simulink model "EricNREL5_FF_Pitch_ConstPwr"  (Simulink 7.7)
settings: Solver=ode4  StartTime=0  StopTime=TMax  FixedStep=DT  MaxStep=DT  RelTol=1e-3
undefined symbols (not defined in the file): alpha, DR, DT, FF_dynamicWindSpeed, FF_Time, GenEff, KI, KK, KP, MaxPit, MinPit, NDOF, NumOuts, OutList, PitDotMax, q_init, qdot_init, SSPitch, strmatch, TdotMax, Tmax, Ts, w_rated, wo
settings Model: Creator=dwilso  LastModifiedBy=oooeee
settings DataIOCC: LimitDataPoints=off  SaveOutput=off  SignalLoggingName=sigsOut
settings OptimizationCC: InlineInvariantSignals=on  InitFltsAndDblsToZero=on
settings DebuggingCC: SaveWithParameterizedLinksMsg=none  SignalResolutionControl=TryResolveAllWithWarning  SolverPrmCheckMsg=none  MultiTaskDSMMsg=warning  MultiTaskCondExecSysMsg=none  StrictBusMsg=None
settings HardwareCC: TargetUnknown=on
settings RTWCC: IncludeERTFirstTime=on
settings GRTTargetCC: TargetFcnLib=ansi_tfl_tmw.mat  ModelReferenceCompliant=off  MatFileLogging=off

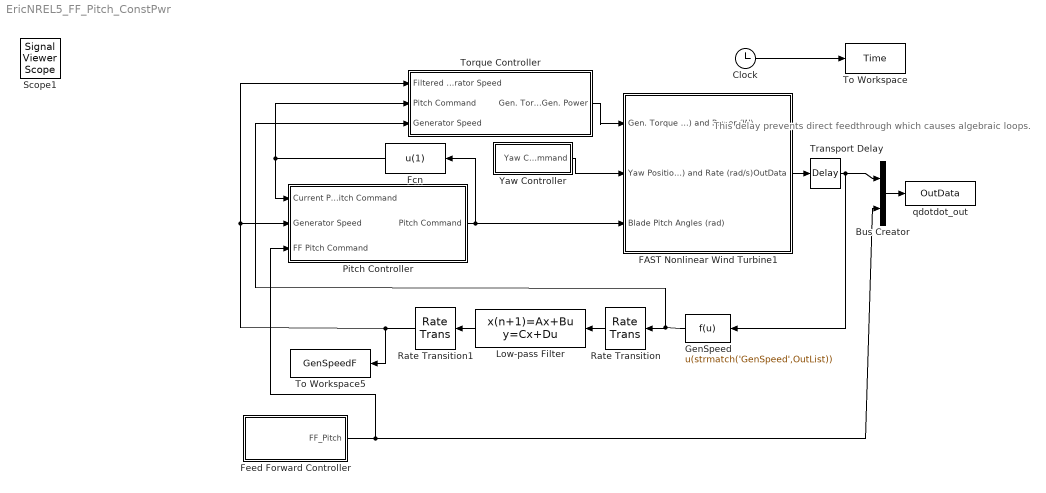
== system EricNREL5_FF_Pitch_ConstPwr ==
  note: This delay prevents direct
      | feedthrough which causes
      |  algebraic loops.
  Bus Creator : BusCreator  Inputs=2
  Clock : Clock
      settings: Decimation=10
  FAST Nonlinear Wind Turbine1 : Subsystem  mask(FAST Nonlinear Wind Turbine){}
      mask help: This block contains the FAST S-Function and blocks that integrate the DOF accelerations to get velocities and displacements.
      mask init:
      | clear FAST_SFunc
  Fcn : Fcn  Expr=u(1)
  Feed Forward Controller : Subsystem
  GenSpeed : Fcn  Expr=u(strmatch('GenSpeed',OutList))
  Low-pass Filter : DiscreteStateSpace  A=alpha  B=1-alpha  C=alpha  D=1-alpha  X0=728.47  SampleTime=Ts
  Pitch Controller : Subsystem
  Rate Transition : RateTransition  OutPortSampleTime=Ts
  Rate Transition1 : RateTransition
  To Workspace : ToWorkspace  VariableName=Time  SampleTime=DT  SaveFormat=Array
  To Workspace5 : ToWorkspace  VariableName=GenSpeedF  SampleTime=-1  SaveFormat=Array
  Torque Controller : Subsystem
  Transport Delay : TransportDelay  DelayTime=.00001
  Yaw Controller : Subsystem
  qdotdot_out : ToWorkspace  VariableName=OutData  SampleTime=DT  SaveFormat=Array
  Scope1 : SignalViewerScope  IOType=viewer  ZoomMode=xonly  RefreshTime=0.035000
  wires:
  Clock/1 -> To Workspace/1
  Yaw Controller/1(Yaw Command) -> FAST Nonlinear Wind Turbine1/2(Yaw Position (rad) and Rate (rad/s))
  GenSpeed/1 -> Rate Transition/1, Torque Controller/3(Generator Speed)
  Low-pass Filter/1 -> Rate Transition1/1
  Fcn/1 -> Pitch Controller/1(Current Pitch Command), Torque Controller/2(Pitch Command)
  Rate Transition/1 -> Low-pass Filter/1
  Rate Transition1/1 -> Torque Controller/1(Filtered Generator Speed), Pitch Controller/2(Generator Speed), To Workspace5/1
  Bus Creator/1 -> qdotdot_out/1
  FAST Nonlinear Wind Turbine1/1(OutData) -> Transport Delay/1
  Transport Delay/1 -> Bus Creator/1, GenSpeed/1
  Torque Controller/1("Gen. Torque,  Gen. Power") -> FAST Nonlinear Wind Turbine1/1(Gen. Torque (Nm) and Power (W))
  Pitch Controller/1(Pitch Command) -> FAST Nonlinear Wind Turbine1/3(Blade Pitch Angles (rad)), Fcn/1
  Feed Forward Controller/1(FF_Pitch) -> Bus Creator/2, Pitch Controller/3(FF Pitch Command)

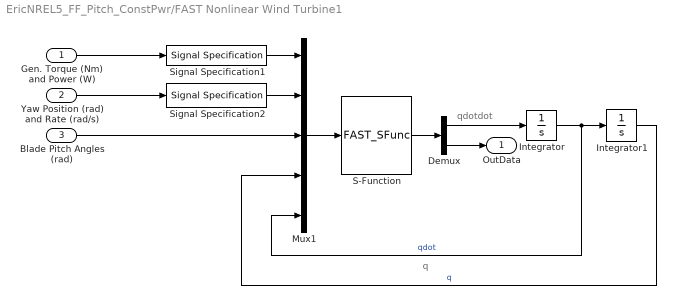
== system EricNREL5_FF_Pitch_ConstPwr/FAST Nonlinear Wind Turbine1 ==
  note: qdotdot
  note: q
  Gen. Torque (Nm) and Power (W) : Inport
  Yaw Position (rad) and Rate (rad/s) : Inport  Port=2
  Blade Pitch Angles (rad) : Inport  Port=3
  Demux : Demux  Outputs=[NDOF, NumOuts]
  Integrator : Integrator  InitialCondition=qdot_init
  Integrator1 : Integrator  InitialCondition=q_init
  Mux1 : Mux  Inputs=5
  S-Function : S-Function  FunctionName=FAST_SFunc  EnableBusSupport=off
  Signal Specification1 : SignalSpecification  OutDataTypeStr=double  Dimensions=2
  Signal Specification2 : SignalSpecification  OutDataTypeStr=double  Dimensions=2
  OutData : Outport
  wires:
  Integrator/1 -> Integrator1/1, Mux1/5  "qdot"
  Gen. Torque (Nm) and Power (W)/1 -> Signal Specification1/1
  S-Function/1 -> Demux/1
  Demux/1 -> Integrator/1
  Demux/2 -> OutData/1
  Mux1/1 -> S-Function/1
  Blade Pitch Angles (rad)/1 -> Mux1/3
  Yaw Position (rad) and Rate (rad/s)/1 -> Signal Specification2/1
  Integrator1/1 -> Mux1/4  "q"
  Signal Specification1/1 -> Mux1/1
  Signal Specification2/1 -> Mux1/2

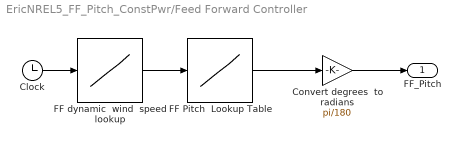
== system EricNREL5_FF_Pitch_ConstPwr/Feed Forward Controller ==
  Clock : Clock
      settings: Decimation=10
  Convert degrees  to radians : Gain  Gain=pi/180
  FF Pitch  Lookup Table : Lookup  InputValues=SSPitch(:,1)  Table=SSPitch(:,2)
  FF dynamic  wind  speed lookup : Lookup  InputValues=FF_Time  Table=FF_dynamicWindSpeed
  FF_Pitch : Outport
  wires:
  FF Pitch  Lookup Table/1 -> Convert degrees  to radians/1
  FF dynamic  wind  speed lookup/1 -> FF Pitch  Lookup Table/1
  Clock/1 -> FF dynamic  wind  speed lookup/1
  Convert degrees  to radians/1 -> FF_Pitch/1

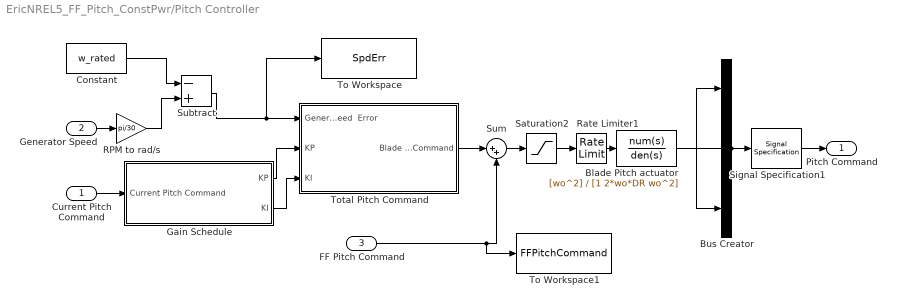
== system EricNREL5_FF_Pitch_ConstPwr/Pitch Controller ==
  Current Pitch Command : Inport
  Generator Speed : Inport  Port=2
  FF Pitch Command : Inport  Port=3
  Blade Pitch actuator : TransferFcn  Numerator=[wo^2]  Denominator=[1 2*wo*DR wo^2]
  Bus Creator : BusCreator  Inputs=3
  Constant : Constant  Value=w_rated
  Gain Schedule : Subsystem
  RPM to rad/s : Gain  Gain=pi/30  SaturateOnIntegerOverflow=on  OutDataTypeStr=Inherit: Same as input  ParamDataTypeStr=Inherit: Same as input
  Rate Limiter1 : RateLimiter  RisingSlewLimit=PitDotMax  FallingSlewLimit=-PitDotMax  SampleTimeMode=inherited
  Saturation2 : Saturate  UpperLimit=MaxPit  LowerLimit=MinPit
  Signal Specification1 : SignalSpecification  OutDataTypeStr=double  Dimensions=3
  Subtract : Sum  Inputs=-+
  Sum : Sum  Inputs=|++
  To Workspace : ToWorkspace  VariableName=SpdErr  SampleTime=-1  SaveFormat=Array
  To Workspace1 : ToWorkspace  VariableName=FFPitchCommand  SampleTime=-1  SaveFormat=Array
  Total Pitch Command : Subsystem
  Pitch Command : Outport
  wires:
  Constant/1 -> Subtract/1
  Bus Creator/1 -> Signal Specification1/1
  Signal Specification1/1 -> Pitch Command/1
  Generator Speed/1 -> RPM to rad/s/1
  Current Pitch Command/1 -> Gain Schedule/1(Current Pitch Command)
  Gain Schedule/1(KP) -> Total Pitch Command/2(KP)
  Gain Schedule/2(KI) -> Total Pitch Command/3(KI)
  Subtract/1 -> Total Pitch Command/1(Generator Speed  Error), To Workspace/1
  RPM to rad/s/1 -> Subtract/2
  Blade Pitch actuator/1 -> Bus Creator/3, Bus Creator/2, Bus Creator/1
  Total Pitch Command/1(Blade Pitch Command) -> Sum/1
  Sum/1 -> Saturation2/1
  FF Pitch Command/1 -> Sum/2, To Workspace1/1
  Saturation2/1 -> Rate Limiter1/1
  Rate Limiter1/1 -> Blade Pitch actuator/1

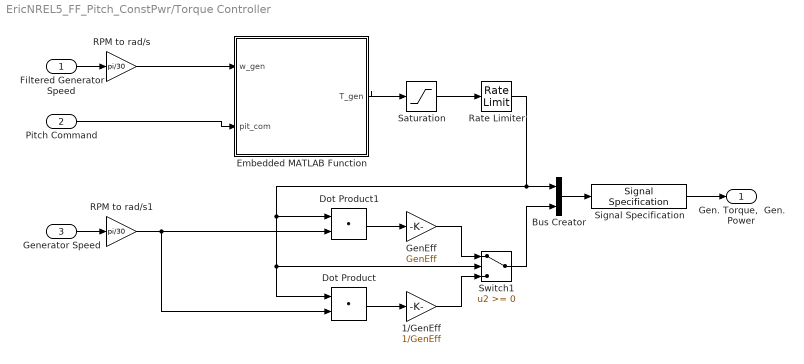
== system EricNREL5_FF_Pitch_ConstPwr/Torque Controller ==
  Filtered Generator Speed : Inport
  Pitch Command : Inport  Port=2
  Generator Speed : Inport  Port=3
  1/GenEff : Gain  Gain=1/GenEff  SaturateOnIntegerOverflow=on  OutDataTypeStr=Inherit: Same as input  ParamDataTypeStr=Inherit: Same as input
  Bus Creator : BusCreator  Inputs=2
  Dot Product : DotProduct  InputSameDT=on  OutDataTypeStr=Inherit: Inherit via internal rule
  Dot Product1 : DotProduct  InputSameDT=on  OutDataTypeStr=Inherit: Inherit via internal rule
  Embedded MATLAB Function : Stateflow chart  TreatAsAtomicUnit=on
  GenEff : Gain  Gain=GenEff  SaturateOnIntegerOverflow=on  OutDataTypeStr=Inherit: Same as input  ParamDataTypeStr=Inherit: Same as input
  RPM to rad/s : Gain  Gain=pi/30  SaturateOnIntegerOverflow=on  OutDataTypeStr=Inherit: Same as input  ParamDataTypeStr=Inherit: Same as input
  RPM to rad/s1 : Gain  Gain=pi/30  SaturateOnIntegerOverflow=on  OutDataTypeStr=Inherit: Same as input  ParamDataTypeStr=Inherit: Same as input
  Rate Limiter : RateLimiter  RisingSlewLimit=TdotMax  FallingSlewLimit=-TdotMax  SampleTimeMode=inherited
  Saturation : Saturate  UpperLimit=Tmax  LowerLimit=0
  Signal Specification : SignalSpecification  OutDataTypeStr=double  Dimensions=2
  Switch1 : Switch  SaturateOnIntegerOverflow=on
  "Gen. Torque,  Gen. Power" : Outport
  wires:
  Embedded MATLAB Function/1(T_gen) -> Saturation/1
  Saturation/1 -> Rate Limiter/1
  Rate Limiter/1 -> Dot Product1/1, Dot Product/1, Switch1/2, Bus Creator/1
  Dot Product/1 -> 1/GenEff/1
  1/GenEff/1 -> Switch1/3
  GenEff/1 -> Switch1/1
  Dot Product1/1 -> GenEff/1
  Switch1/1 -> Bus Creator/2
  Pitch Command/1 -> Embedded MATLAB Function/2(pit_com)
  Signal Specification/1 -> "Gen. Torque,  Gen. Power"/1
  Bus Creator/1 -> Signal Specification/1
  RPM to rad/s/1 -> Embedded MATLAB Function/1(w_gen)
  Filtered Generator Speed/1 -> RPM to rad/s/1
  Generator Speed/1 -> RPM to rad/s1/1
  RPM to rad/s1/1 -> Dot Product1/2, Dot Product/2

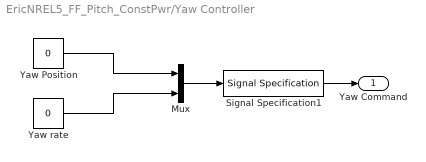
== system EricNREL5_FF_Pitch_ConstPwr/Yaw Controller ==
  Mux : Mux  Inputs=2
  Signal Specification1 : SignalSpecification  OutDataTypeStr=double  Dimensions=2
  Yaw Position : Constant  Value=0
  Yaw rate : Constant  Value=0
  Yaw Command : Outport
  wires:
  Mux/1 -> Signal Specification1/1
  Yaw Position/1 -> Mux/1
  Yaw rate/1 -> Mux/2
  Signal Specification1/1 -> Yaw Command/1

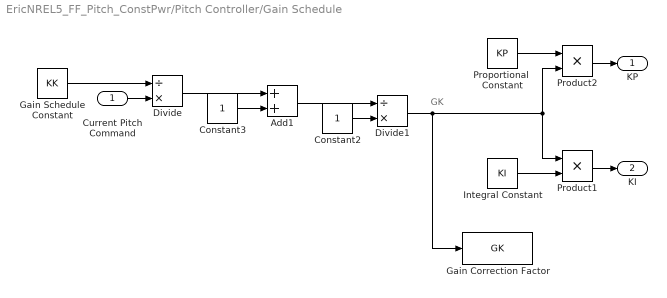
== system EricNREL5_FF_Pitch_ConstPwr/Pitch Controller/Gain Schedule ==
  note: GK
  Current Pitch Command : Inport
  Add1 : Sum
  Constant2 : Constant
  Constant3 : Constant
  Divide : Product  Inputs=/*
  Divide1 : Product  Inputs=/*
  Gain Schedule Constant : Constant  Value=KK
  Gain Correction Factor : ToWorkspace  VariableName=GK  SampleTime=-1  SaveFormat=Array
  Integral Constant : Constant  Value=KI
  Product1 : Product  RndMeth=Zero
  Product2 : Product  RndMeth=Zero
  Proportional  Constant : Constant  Value=KP
  KP : Outport
  KI : Outport  Port=2
  wires:
  Constant2/1 -> Divide1/2
  Add1/1 -> Divide1/1
  Constant3/1 -> Add1/2
  Divide/1 -> Add1/1
  Gain Schedule Constant/1 -> Divide/1
  Divide1/1 -> Product2/2, Product1/1, Gain Correction Factor/1
  Proportional  Constant/1 -> Product2/1
  Integral Constant/1 -> Product1/2
  Product2/1 -> KP/1
  Current Pitch Command/1 -> Divide/2
  Product1/1 -> KI/1

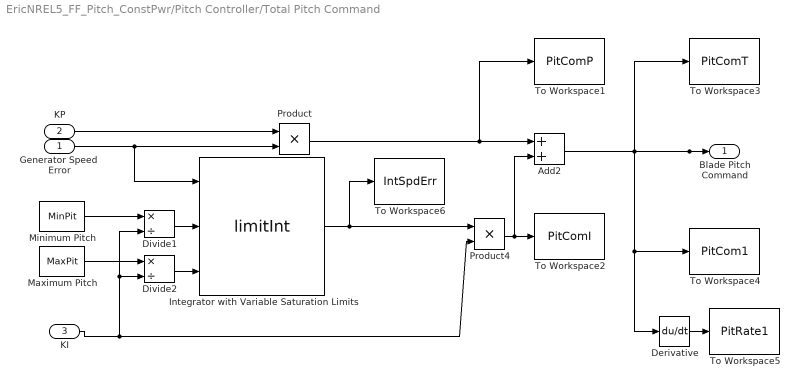
== system EricNREL5_FF_Pitch_ConstPwr/Pitch Controller/Total Pitch Command ==
  Generator Speed  Error : Inport
  KP : Inport  Port=2
  KI : Inport  Port=3
  Add2 : Sum
  Derivative : Derivative
  Divide1 : Product  Inputs=*/
  Divide2 : Product  Inputs=*/
  Integrator with Variable Saturation Limits : M-S-Function  FunctionName=limitInt  Parameters=xi  mask{xi=0}
      mask prompts: xi "Initial Condition"
      mask Display:
      | disp('1\n-----\ns')
      | port_label('input',2,'LB')
      | port_label('input',3,'UB')
  Maximum Pitch : Constant  Value=MaxPit
  Minimum Pitch : Constant  Value=MinPit
  Product : Product  RndMeth=Zero
  Product4 : Product  RndMeth=Zero
  To Workspace1 : ToWorkspace  VariableName=PitComP  SampleTime=-1  SaveFormat=Array
  To Workspace2 : ToWorkspace  VariableName=PitComI  SampleTime=-1  SaveFormat=Array
  To Workspace3 : ToWorkspace  VariableName=PitComT  SampleTime=-1  SaveFormat=Array
  To Workspace4 : ToWorkspace  VariableName=PitCom1  SampleTime=-1  SaveFormat=Array
  To Workspace5 : ToWorkspace  VariableName=PitRate1  SampleTime=-1  SaveFormat=Array
  To Workspace6 : ToWorkspace  VariableName=IntSpdErr  SampleTime=-1  SaveFormat=Array
  Blade Pitch Command : Outport
  wires:
  Generator Speed  Error/1 -> Product/2, Integrator with Variable Saturation Limits/1
  Product/1 -> Add2/1, To Workspace1/1
  Product4/1 -> Add2/2, To Workspace2/1
  KP/1 -> Product/1
  KI/1 -> Product4/2, Divide1/2, Divide2/2
  Maximum Pitch/1 -> Divide2/1
  Derivative/1 -> To Workspace5/1
  Minimum Pitch/1 -> Divide1/1
  Divide1/1 -> Integrator with Variable Saturation Limits/2
  Divide2/1 -> Integrator with Variable Saturation Limits/3
  Integrator with Variable Saturation Limits/1 -> Product4/1, To Workspace6/1
  Add2/1 -> To Workspace3/1, Blade Pitch Command/1, To Workspace4/1, Derivative/1

== matlab function Torque Controller/Embedded MATLAB Function ==
  data: w_gen input double; T_gen output double; pit_com input double
function T_gen = GenTorque(w_gen,pit_com)

%Set up all of the torque controller constants
w_cutin = 70.16224; %rad/s
w_rated = 121.6805; %rad/s
k_gen = 2.332287; %(N-m)/(rad/s)^2
P_max = 5296610.0; %Watts

m15 = (1.3*w_cutin)^2*k_gen/(1.3*w_cutin-w_cutin); %Region 1.5 Slope
m25 = (P_max/w_rated)/(w_rated-w_rated/1.1); %Region 2.5 slope
w_sysp = w_rated/1.1; %speed where the turbine operates as a synchronous induction generator  
w_TrGen = (m25-sqrt(m25^2-4*k_gen*w_sysp*m25))/(2*k_gen); %Transition speed from region 2 to region 2.5
minPit3 = 1*pi/180; %Minimum pitch angle command that puts the turbine into region 3

if w_gen < w_cutin
	T_gen = 0;
elseif w_gen < 1.3*w_cutin
	T_gen = m15*(w_gen-w_cutin);
elseif w_gen < w_TrGen
	T_gen = k_gen*w_gen^2;
elseif w_gen < w_rated
	T_gen = m25*(w_gen-w_sysp);
else 
    T_gen = P_max/w_gen;
end

if pit_com >= minPit3
    T_gen = P_max/w_gen;
end
